simulink model "HUAUV3_"  (R2019a)
settings: Solver=VariableStepAuto  StartTime=0.0  StopTime=30  RelTol=1e-3
InitFcn:
  | run('HUAUVInitial.m')
values from neighbouring files (symbols this model uses):
  buoPos =     [HUAUVPARAMETERS.mat]
  coeff =     [HUAUVPARAMETERS.mat]
  g = 9.8    [HUAUVInitial.m]    (also in HUAUVPARAMETERS.mat)
  Jx = 2.365e-2    (= 0.02365)    [HUAUVInitial.m]    (also in HUAUVPARAMETERS.mat)
  Jy = 1.318e-2    (= 0.01318)    [HUAUVInitial.m]    (also in HUAUVPARAMETERS.mat)
  Jz = 1.318e-2    (= 0.01318)    [HUAUVInitial.m]    (also in HUAUVPARAMETERS.mat)
  m = 1.8    [HUAUVInitial.m]    (also in HUAUVPARAMETERS.mat)
  Sx = 0.07*0.15    (= 0.0105)    [HUAUVInitial.m]    (also in HUAUVPARAMETERS.mat)
  Sy = 0.07*0.28    (= 0.0196)    [HUAUVInitial.m]    (also in HUAUVPARAMETERS.mat)
  Sz = 0.15*0.28    (= 0.042)    [HUAUVInitial.m]    (also in HUAUVPARAMETERS.mat)
  V = 1e-3    (= 0.001)    [HUAUVInitial.m]
undefined symbols (not defined in the file or in its folder): rho
libraries: simulink x12, shared6dof x2
(part 2 of 2)

== system HUAUV3_/HUAUV  MODEL/UNDERWATER MODEL/position PID controller1 ==
  targetPositions : Inport
  realPosition : Inport  Port=2
  Demux : Demux  Outputs=3
  Demux1 : Demux  Outputs=3
  Mux : Mux  Inputs=3
  Saturation : Saturate  UpperLimit=100  LowerLimit=-100
  Saturation1 : Saturate  UpperLimit=100  LowerLimit=-100
  Saturation2 : Saturate  UpperLimit=200  LowerLimit=-200
  Sum : Sum  Inputs=+-
  Sum1 : Sum  Inputs=+-
  Sum2 : Sum  Inputs=+-
  x : simulink/Continuous/PID Controller  Controller=PID  Form=Parallel  TimeDomain=Continuous-time  SampleTime=-1  IntegratorMethod=Forward Euler  FilterMethod=Forward Euler  ControllerParametersSource=internal  P=150  I=70  D=80  UseFilter=on  N=9099.36023942606  TunerSelectOption=Transfer Function Based (PID Tuner App)  InitialConditionSource=internal  InitialConditionForIntegrator=0  InitialConditionForFilter=0  DifferentiatorICPrevScaledInput=0  ExternalReset=none  TrackingMode=off  Kt=1  LimitOutput=off  UpperSaturationLimit=inf  LowerSaturationLimit=-inf  LinearizeAsGain=on  AntiWindupMode=none  Kb=1  POutMin=[]  POutMax=[]  IOutMin=[]  IOutMax=[]  DOutMin=[]  DOutMax=[]  NOutMin=[]  NOutMax=[]  SumOutMin=[]  SumOutMax=[]  SaturationOutMin=[]  SaturationOutMax=[]  PParamMin=[]  PParamMax=[]  IParamMin=[]  IParamMax=[]  DParamMin=[]  DParamMax=[]  NParamMin=[]  NParamMax=[]  KbParamMin=[]  KbParamMax=[]  KtParamMin=[]  KtParamMax=[]  KbOutMin=[]  KbOutMax=[]  KtOutMin=[]  KtOutMax=[]  IntegratorOutMin=[]  IntegratorOutMax=[]  FilterOutMin=[]  FilterOutMax=[]  SumI1OutMin=[]  SumI1OutMax=[]  SumI2OutMin=[]  SumI2OutMax=[]  SumI3OutMin=[]  SumI3OutMax=[]  SumI4OutMin=[]  SumI4OutMax=[]  SumDOutMin=[]  SumDOutMax=[]  DifferentiatorOutMin=[]  DifferentiatorOutMax=[]  FilterDiffOutCoefMin=[]  FilterDiffOutCoefMax=[]  ReciprocalOutMin=[]  ReciprocalOutMax=[]  SumDenOutMin=[]  SumDenOutMax=[]  SumNumOutMin=[]  SumNumOutMax=[]  DivideOutMin=[]  DivideOutMax=[]  IntegratorContinuousStateAttributes=''  IntegratorStateMustResolveToSignalObject=off  IntegratorRTWStateStorageClass=Auto  FilterContinuousStateAttributes=''  FilterStateMustResolveToSignalObject=off  FilterRTWStateStorageClass=Auto  ParallelPVariant=InternalParameters  IdealPVariant=Disabled  IVariant=InternalParameters  DVariant=InternalParameters  IntegratorVariant=Continuous  SatVariant=Disabled  AWVariant=Passthrough  PCopyVariant=Disabled  TRVariant=Disabled  FdbkBlocksVariant=Forward  IdealPFdbkVariant=Disabled  SatFdbkVariant=Disabled  DerivativeFilterVariant=ContFilter  NVariant=InternalParameters  NCopyVariant=Disabled  FilterICVariant=InternalICsFilter  IntegratorICVariant=InternalICs  ExternalResetVariant=Disabled  TRSumVariant=Passthrough  SumFdbkVariant=Disabled  SumVariant=Sum_PID
  y : simulink/Continuous/PID Controller  Controller=PID  Form=Parallel  TimeDomain=Continuous-time  SampleTime=-1  IntegratorMethod=Forward Euler  FilterMethod=Forward Euler  ControllerParametersSource=internal  P=36.8420392063011  I=3.4  D=51.7115453208585  UseFilter=on  N=1442.15140992177  TunerSelectOption=Transfer Function Based (PID Tuner App)  InitialConditionSource=internal  InitialConditionForIntegrator=0  InitialConditionForFilter=0  DifferentiatorICPrevScaledInput=0  ExternalReset=none  TrackingMode=off  Kt=1  LimitOutput=off  UpperSaturationLimit=inf  LowerSaturationLimit=-inf  LinearizeAsGain=on  AntiWindupMode=none  Kb=1  POutMin=[]  POutMax=[]  IOutMin=[]  IOutMax=[]  DOutMin=[]  DOutMax=[]  NOutMin=[]  NOutMax=[]  SumOutMin=[]  SumOutMax=[]  SaturationOutMin=[]  SaturationOutMax=[]  PParamMin=[]  PParamMax=[]  IParamMin=[]  IParamMax=[]  DParamMin=[]  DParamMax=[]  NParamMin=[]  NParamMax=[]  KbParamMin=[]  KbParamMax=[]  KtParamMin=[]  KtParamMax=[]  KbOutMin=[]  KbOutMax=[]  KtOutMin=[]  KtOutMax=[]  IntegratorOutMin=[]  IntegratorOutMax=[]  FilterOutMin=[]  FilterOutMax=[]  SumI1OutMin=[]  SumI1OutMax=[]  SumI2OutMin=[]  SumI2OutMax=[]  SumI3OutMin=[]  SumI3OutMax=[]  SumI4OutMin=[]  SumI4OutMax=[]  SumDOutMin=[]  SumDOutMax=[]  DifferentiatorOutMin=[]  DifferentiatorOutMax=[]  FilterDiffOutCoefMin=[]  FilterDiffOutCoefMax=[]  ReciprocalOutMin=[]  ReciprocalOutMax=[]  SumDenOutMin=[]  SumDenOutMax=[]  SumNumOutMin=[]  SumNumOutMax=[]  DivideOutMin=[]  DivideOutMax=[]  IntegratorContinuousStateAttributes=''  IntegratorStateMustResolveToSignalObject=off  IntegratorRTWStateStorageClass=Auto  FilterContinuousStateAttributes=''  FilterStateMustResolveToSignalObject=off  FilterRTWStateStorageClass=Auto  ParallelPVariant=InternalParameters  IdealPVariant=Disabled  IVariant=InternalParameters  DVariant=InternalParameters  IntegratorVariant=Continuous  SatVariant=Disabled  AWVariant=Passthrough  PCopyVariant=Disabled  TRVariant=Disabled  FdbkBlocksVariant=Forward  IdealPFdbkVariant=Disabled  SatFdbkVariant=Disabled  DerivativeFilterVariant=ContFilter  NVariant=InternalParameters  NCopyVariant=Disabled  FilterICVariant=InternalICsFilter  IntegratorICVariant=InternalICs  ExternalResetVariant=Disabled  TRSumVariant=Passthrough  SumFdbkVariant=Disabled  SumVariant=Sum_PID
  z : simulink/Continuous/PID Controller  Controller=PID  Form=Parallel  TimeDomain=Continuous-time  SampleTime=-1  IntegratorMethod=Forward Euler  FilterMethod=Forward Euler  ControllerParametersSource=internal  P=59  I=10  D=71.2928934671724  UseFilter=on  N=3622.5205587649  TunerSelectOption=Transfer Function Based (PID Tuner App)  InitialConditionSource=internal  InitialConditionForIntegrator=0  InitialConditionForFilter=0  DifferentiatorICPrevScaledInput=0  ExternalReset=none  TrackingMode=off  Kt=1  LimitOutput=off  UpperSaturationLimit=inf  LowerSaturationLimit=-inf  LinearizeAsGain=on  AntiWindupMode=none  Kb=1  POutMin=[]  POutMax=[]  IOutMin=[]  IOutMax=[]  DOutMin=[]  DOutMax=[]  NOutMin=[]  NOutMax=[]  SumOutMin=[]  SumOutMax=[]  SaturationOutMin=[]  SaturationOutMax=[]  PParamMin=[]  PParamMax=[]  IParamMin=[]  IParamMax=[]  DParamMin=[]  DParamMax=[]  NParamMin=[]  NParamMax=[]  KbParamMin=[]  KbParamMax=[]  KtParamMin=[]  KtParamMax=[]  KbOutMin=[]  KbOutMax=[]  KtOutMin=[]  KtOutMax=[]  IntegratorOutMin=[]  IntegratorOutMax=[]  FilterOutMin=[]  FilterOutMax=[]  SumI1OutMin=[]  SumI1OutMax=[]  SumI2OutMin=[]  SumI2OutMax=[]  SumI3OutMin=[]  SumI3OutMax=[]  SumI4OutMin=[]  SumI4OutMax=[]  SumDOutMin=[]  SumDOutMax=[]  DifferentiatorOutMin=[]  DifferentiatorOutMax=[]  FilterDiffOutCoefMin=[]  FilterDiffOutCoefMax=[]  ReciprocalOutMin=[]  ReciprocalOutMax=[]  SumDenOutMin=[]  SumDenOutMax=[]  SumNumOutMin=[]  SumNumOutMax=[]  DivideOutMin=[]  DivideOutMax=[]  IntegratorContinuousStateAttributes=''  IntegratorStateMustResolveToSignalObject=off  IntegratorRTWStateStorageClass=Auto  FilterContinuousStateAttributes=''  FilterStateMustResolveToSignalObject=off  FilterRTWStateStorageClass=Auto  ParallelPVariant=InternalParameters  IdealPVariant=Disabled  IVariant=InternalParameters  DVariant=InternalParameters  IntegratorVariant=Continuous  SatVariant=Disabled  AWVariant=Passthrough  PCopyVariant=Disabled  TRVariant=Disabled  FdbkBlocksVariant=Forward  IdealPFdbkVariant=Disabled  SatFdbkVariant=Disabled  DerivativeFilterVariant=ContFilter  NVariant=InternalParameters  NCopyVariant=Disabled  FilterICVariant=InternalICsFilter  IntegratorICVariant=InternalICs  ExternalResetVariant=Disabled  TRSumVariant=Passthrough  SumFdbkVariant=Disabled  SumVariant=Sum_PID
  posControlOut : Outport
  wires:
  Sum1/1 -> y/1
  y/1 -> Saturation1/1
  Demux1/2 -> Sum1/2
  Demux/3 -> Sum2/1
  Demux/2 -> Sum1/1
  Demux/1 -> Sum/1
  Sum/1 -> x/1
  z/1 -> Saturation2/1
  Sum2/1 -> z/1
  Demux1/3 -> Sum2/2
  targetPositions/1 -> Demux/1
  realPosition/1 -> Demux1/1
  Mux/1 -> posControlOut/1
  x/1 -> Saturation/1
  Saturation/1 -> Mux/1
  Saturation1/1 -> Mux/2
  Saturation2/1 -> Mux/3
  Demux1/1 -> Sum/2

== system HUAUV3_/HUAUV  MODEL/AIR MODEL/HUAUV AIR MODEL/frame parameters ==
  Constant : Constant  Value=m
  J : Constant  Value=[Jx Jy Jz]
  to dialog matrix : Subsystem
  zeros(3x3) : Constant  Value=zeros(3,3)
  m : Outport
  dI/dt : Outport  Port=2
  I : Outport  Port=3
  wires:
  J/1 -> to dialog matrix/1(3 element vector)
  zeros(3x3)/1 -> dI/dt/1
  Constant/1 -> m/1
  to dialog matrix/1(matrix) -> I/1

== system HUAUV3_/HUAUV  MODEL/UNDERWATER MODEL/HUAUV UNDERWATER MODEL/frame parameters ==
  Constant : Constant  Value=m+2.25
  J : Constant  Value=[Jx+5e-2 Jy+5e-2 Jz+1e-1]
  to dialog matrix : Subsystem
  zeros(3x3) : Constant  Value=zeros(3,3)
  m : Outport
  dI/dt : Outport  Port=2
  I : Outport  Port=3
  wires:
  J/1 -> to dialog matrix/1(3 element vector)
  zeros(3x3)/1 -> dI/dt/1
  Constant/1 -> m/1
  to dialog matrix/1(matrix) -> I/1

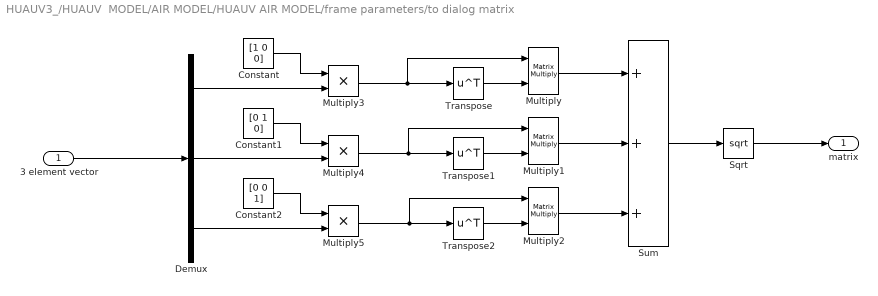
== system HUAUV3_/HUAUV  MODEL/AIR MODEL/HUAUV AIR MODEL/frame parameters/to dialog matrix ==
  3 element vector : Inport
  Constant : Constant  Value=[1 0 0]
  Constant1 : Constant  Value=[0 1 0]
  Constant2 : Constant  Value=[0 0 1]
  Demux : Demux  Outputs=3
  Multiply : Product  Multiplication=Matrix(*)
  Multiply1 : Product  Multiplication=Matrix(*)
  Multiply2 : Product  Multiplication=Matrix(*)
  Multiply3 : Product
  Multiply4 : Product
  Multiply5 : Product
  Sqrt : Sqrt  SaturateOnIntegerOverflow=on
  Sum : Sum  Inputs=+++
  Transpose : Math  Operator=transpose  SaturateOnIntegerOverflow=on
  Transpose1 : Math  Operator=transpose  SaturateOnIntegerOverflow=on
  Transpose2 : Math  Operator=transpose  SaturateOnIntegerOverflow=on
  matrix : Outport
  wires:
  Sum/1 -> Sqrt/1
  3 element vector/1 -> Demux/1
  Multiply1/1 -> Sum/2
  Multiply/1 -> Sum/1
  Multiply2/1 -> Sum/3
  Demux/1 -> Multiply3/2
  Demux/2 -> Multiply4/2
  Demux/3 -> Multiply5/2
  Constant/1 -> Multiply3/1
  Multiply3/1 -> Multiply/1, Transpose/1
  Constant1/1 -> Multiply4/1
  Constant2/1 -> Multiply5/1
  Multiply4/1 -> Multiply1/1, Transpose1/1
  Transpose/1 -> Multiply/2
  Transpose1/1 -> Multiply1/2
  Transpose2/1 -> Multiply2/2
  Multiply5/1 -> Transpose2/1, Multiply2/1
  Sqrt/1 -> matrix/1

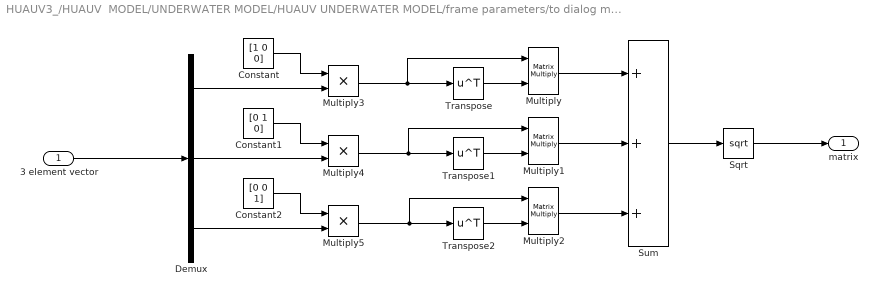
== system HUAUV3_/HUAUV  MODEL/UNDERWATER MODEL/HUAUV UNDERWATER MODEL/frame parameters/to dialog matrix ==
  3 element vector : Inport
  Constant : Constant  Value=[1 0 0]
  Constant1 : Constant  Value=[0 1 0]
  Constant2 : Constant  Value=[0 0 1]
  Demux : Demux  Outputs=3
  Multiply : Product  Multiplication=Matrix(*)
  Multiply1 : Product  Multiplication=Matrix(*)
  Multiply2 : Product  Multiplication=Matrix(*)
  Multiply3 : Product
  Multiply4 : Product
  Multiply5 : Product
  Sqrt : Sqrt  SaturateOnIntegerOverflow=on
  Sum : Sum  Inputs=+++
  Transpose : Math  Operator=transpose  SaturateOnIntegerOverflow=on
  Transpose1 : Math  Operator=transpose  SaturateOnIntegerOverflow=on
  Transpose2 : Math  Operator=transpose  SaturateOnIntegerOverflow=on
  matrix : Outport
  wires:
  Sum/1 -> Sqrt/1
  3 element vector/1 -> Demux/1
  Multiply1/1 -> Sum/2
  Multiply/1 -> Sum/1
  Multiply2/1 -> Sum/3
  Demux/1 -> Multiply3/2
  Demux/2 -> Multiply4/2
  Demux/3 -> Multiply5/2
  Constant/1 -> Multiply3/1
  Multiply3/1 -> Multiply/1, Transpose/1
  Constant1/1 -> Multiply4/1
  Constant2/1 -> Multiply5/1
  Multiply4/1 -> Multiply1/1, Transpose1/1
  Transpose/1 -> Multiply/2
  Transpose1/1 -> Multiply1/2
  Transpose2/1 -> Multiply2/2
  Multiply5/1 -> Transpose2/1, Multiply2/1
  Sqrt/1 -> matrix/1
